simulink model "spill_controller_relative"  (Simulink 4.00)
settings: Solver=ode45  SolverMode=SingleTasking  StartTime=0.0  StopTime=0.04  FixedStep=0.0000001  RelTol=1e-3
undefined symbols (not defined in the file): K_s, miu_A_spill, Valve_time
settings Model: Creator=mandic  LastModifiedBy=CAIKA  LoadExternalInput=on  ExternalInput=[u]  RTWOptions="-aEnforceIntegerDowncast=1 -aExtMode=0 -aFoldNonRolledExpr=1 -aForceParamTrailComments=0 -aGenerateComments=1 -aIgnoreCustomStorageClasses=0 -aIncHierarchyInIds=0 -aInlineInvariantSignals=0 -aInlineParameters=0 -aLocalBlockOutputs=1 -aLogVarNameModifier=\"rt_\" -aRTWVerbose=1 -aRollThreshold=5 -aShowEliminatedStatements=1"  RTWRetainRTWFile=on  RTWTemplateMakefile=avl_grt_dll_nt.tmf  RTWMakeCommand=make_rtw PROGRAM=hy_pid  ExtModeTrigMode=oneshot  ExtModeArmWhenConnect=off

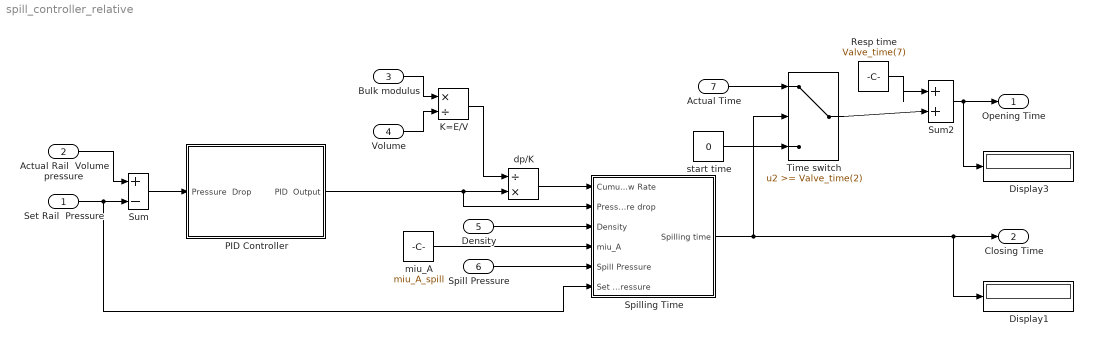
== system spill_controller_relative ==
  Set Rail  Pressure : Inport  Port=1  LatchInput=off
  Actual Rail  Volume pressure : Inport  Port=2  LatchInput=off
  Bulk modulus : Inport  Port=3  LatchInput=off
  Volume : Inport  Port=4  LatchInput=off
  Density : Inport  Port=5  LatchInput=off
  Spill Pressure : Inport  Port=6  LatchInput=off
  Actual Time : Inport  Port=7  LatchInput=off
  Display1 : Display
      settings: Format=short_e
  Display3 : Display
      settings: Format=short_e
  K=E/V : Product  Inputs=*/  Multiplication=Element-wise(.*)  SaturateOnIntegerOverflow=on
  PID Controller : Subsystem
      settings: RTWFcnNameOpts=Auto  RTWFileNameOpts=Auto
  Resp time : Constant  Value=Valve_time(7)
  Spilling Time : Subsystem
      settings: RTWFcnNameOpts=Auto  RTWFileNameOpts=Auto
  Sum : Sum  Inputs=|+-  SaturateOnIntegerOverflow=on
  Sum2 : Sum  Inputs=|++  SaturateOnIntegerOverflow=on
  Time switch : Switch  Threshold=Valve_time(2)
  dp/K : Product  Inputs=/*  Multiplication=Element-wise(.*)  SaturateOnIntegerOverflow=on
  miu_A : Constant  Value=miu_A_spill
  start time : Constant  Value=0
  Opening Time : Outport  Port=1
  Closing Time : Outport  Port=2
  wires:
  PID Controller/1(PID  Output) -> dp/K/2, Spilling Time/2(Pressure drop)
  Bulk modulus/1 -> K=E/V/1
  Volume/1 -> K=E/V/2
  K=E/V/1 -> dp/K/1
  dp/K/1 -> Spilling Time/1(Cumulative  Flow Rate)
  Density/1 -> Spilling Time/3(Density)
  miu_A/1 -> Spilling Time/4(miu_A)
  Spilling Time/1(Spilling time) -> Time switch/2, Closing Time/1, Display1/1
  Actual Rail  Volume pressure/1 -> Sum/1
  Set Rail  Pressure/1 -> Sum/2, Spilling Time/6(Set Rail  Pressure)
  Spill Pressure/1 -> Spilling Time/5(Spill Pressure)
  start time/1 -> Time switch/3
  Actual Time/1 -> Time switch/1
  Sum/1 -> PID Controller/1(Pressure  Drop)
  Resp time/1 -> Sum2/1
  Sum2/1 -> Opening Time/1, Display3/1
  Time switch/1 -> Sum2/2

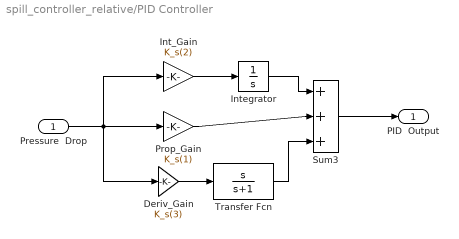
== system spill_controller_relative/PID Controller ==
  Pressure  Drop : Inport  Port=1  LatchInput=off
  Deriv_Gain : Gain  Gain=K_s(3)  Multiplication=Element-wise(K.*u)  SaturateOnIntegerOverflow=on
  Int_Gain : Gain  Gain=K_s(2)  Multiplication=Element-wise(K.*u)  SaturateOnIntegerOverflow=on
  Integrator : Integrator  ExternalReset=none  InitialConditionSource=internal  InitialCondition=0  LimitOutput=off  UpperSaturationLimit=inf  LowerSaturationLimit=-inf  ShowSaturationPort=off  ShowStatePort=off  AbsoluteTolerance=auto
  Prop_Gain : Gain  Gain=K_s(1)  Multiplication=Element-wise(K.*u)  SaturateOnIntegerOverflow=on
  Sum3 : Sum  Inputs=|+++  SaturateOnIntegerOverflow=on
  Transfer Fcn : TransferFcn  Numerator=[1 0]  Denominator=[1 1]  AbsoluteTolerance=auto  Realization=auto
  PID  Output : Outport  Port=1
  wires:
  Int_Gain/1 -> Integrator/1
  Prop_Gain/1 -> Sum3/2
  Integrator/1 -> Sum3/1
  Transfer Fcn/1 -> Sum3/3
  Deriv_Gain/1 -> Transfer Fcn/1
  Pressure  Drop/1 -> Prop_Gain/1, Int_Gain/1, Deriv_Gain/1
  Sum3/1 -> PID  Output/1

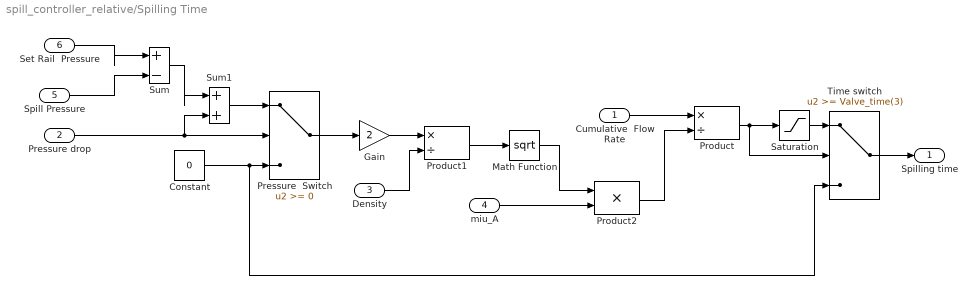
== system spill_controller_relative/Spilling Time ==
  Cumulative  Flow Rate : Inport  Port=1  LatchInput=off
  Pressure drop : Inport  Port=2  LatchInput=off
  Density : Inport  Port=3  LatchInput=off
  miu_A : Inport  Port=4  LatchInput=off
  Spill Pressure : Inport  Port=5  LatchInput=off
  Set Rail  Pressure : Inport  Port=6  LatchInput=off
  Constant : Constant  Value=0
  Gain : Gain  Gain=2  Multiplication=Element-wise(K.*u)  SaturateOnIntegerOverflow=on
  Math Function : Math  Operator=sqrt  OutputSignalType=auto
  Pressure  Switch : Switch  Threshold=0
  Product : Product  Inputs=*/  Multiplication=Element-wise(.*)  SaturateOnIntegerOverflow=on
  Product1 : Product  Inputs=*/  Multiplication=Element-wise(.*)  SaturateOnIntegerOverflow=on
  Product2 : Product  Inputs=2  Multiplication=Element-wise(.*)  SaturateOnIntegerOverflow=on
  Saturation : Saturate  UpperLimit=Valve_time(1)-(Valve_time(4)+Valve_time(6))  LowerLimit=Valve_time(3)+Valve_time(5)  LinearizeAsGain=on
  Sum : Sum  Inputs=|+-  SaturateOnIntegerOverflow=on
  Sum1 : Sum  Inputs=|++  SaturateOnIntegerOverflow=on
  Time switch : Switch  Threshold=Valve_time(3)
  Spilling time : Outport  Port=1
  wires:
  Gain/1 -> Product1/1
  Density/1 -> Product1/2
  Product1/1 -> Math Function/1
  Math Function/1 -> Product2/1
  miu_A/1 -> Product2/2
  Cumulative  Flow Rate/1 -> Product/1
  Product2/1 -> Product/2
  Constant/1 -> Pressure  Switch/3, Time switch/3
  Pressure  Switch/1 -> Gain/1
  Product/1 -> Saturation/1, Time switch/2
  Pressure drop/1 -> Pressure  Switch/2, Sum1/2
  Set Rail  Pressure/1 -> Sum/1
  Spill Pressure/1 -> Sum/2
  Sum/1 -> Sum1/1
  Sum1/1 -> Pressure  Switch/1
  Saturation/1 -> Time switch/1
  Time switch/1 -> Spilling time/1
